simulink model "ThreeDOF_Rocket_Simulator_v2"  (R2023b)
settings: Solver=VariableStepAuto  StartTime=0.0  StopTime=100  RelTol=1e-3
libraries: shared3dof x1, simulink x1
settings Model: PacingRate=0.500000  Creator=giuse  LastModifiedBy=giuse
settings OptimizationCC: ReuseModelBlockBuffer=off
settings DebuggingCC: UnconnectedInputMsg=warning  UnconnectedOutputMsg=warning  UnconnectedLineMsg=warning
settings ModelReferenceCC: EnableRefExpFcnMdlSchedulingChecks=on
settings RTWCC: DLArmComputeVersion=19.05

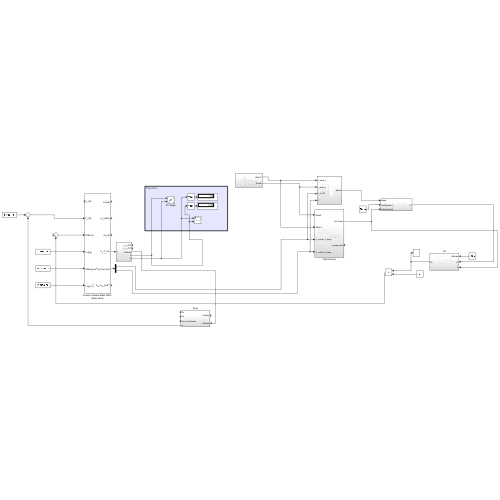
[thumbnail: Simulink's stored preview of the top-level diagram]
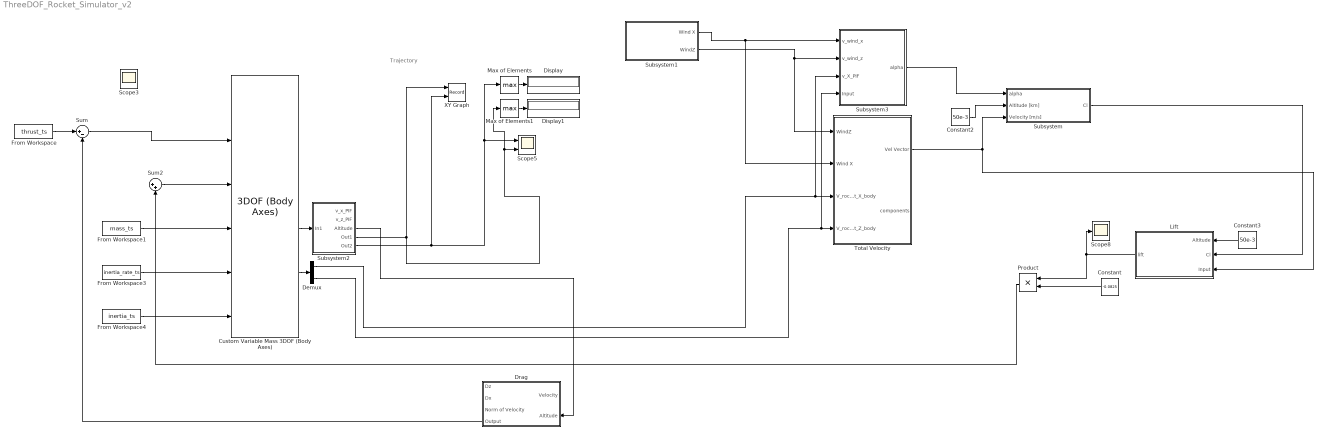
== system ThreeDOF_Rocket_Simulator_v2 ==
  note: Trajectory
  Constant : Constant  Value=-0.0825  VectorParams1D=off
  Constant2 : Constant  Value=50e-3
  Constant3 : Constant  Value=50e-3
  Custom Variable Mass 3DOF (Body Axes) : shared3dof/3DOF (Body Axes)  units=Metric (MKS)  mtype=Custom Variable  v_ini=0  theta_ini=pi  alpha_ini=pi/2  pos_ini=[0 0]  q_ini=0  mass=1.0  mass_e=0.5  mass_f=3.0  Iyy=1.0  Iyy_e=0.5  Iyy_f=3.0  g_in=Internal  g=9.81  vre_flag=off  abi_flag=off  aMode=0  vel_statename=''  theta_statename=''  pos_statename=''  q_statename=''  mass_statename=''
  Demux : Demux  Outputs=2
  Display : Display
  Display1 : Display
  Drag : Subsystem
  From Workspace : FromWorkspace  VariableName=thrust_ts
  From Workspace1 : FromWorkspace  VariableName=mass_ts
  From Workspace3 : FromWorkspace  VariableName=inertia_rate_ts
  From Workspace4 : FromWorkspace  VariableName=inertia_ts
  Lift : Subsystem
  Max of Elements : MinMax  Function=max
  Max of Elements1 : MinMax  Function=max
  Product : Product
  Scope5 : Scope  NumInputPorts=2
  Scope8 : Scope
  Subsystem : Subsystem
  Subsystem1 : Subsystem
  Subsystem2 : Subsystem
  Subsystem3 : Subsystem
  Sum : Sum  Inputs=|+-
  Sum2 : Sum  Inputs=|++
  Total Velocity : Subsystem
  XY Graph : Record  FileSettingsInternal="{\"entries\":[{\"content\":{\"excelSettings\":{\"content\":{},\"type\":\"Streamout.ExcelSettings\"}},\"type\":\"Streamout.FileSettingStorage\",\"uuid\":\"\"}],\"packageUris\":[\"http:\\/\\/schema.mathworks.com\\/mf0\\/streamout_blocks\\/R2020a\"],\"version\":\"1.0\"}"  Layout=[1 1]  SignalsInternal="{\"entries\":[{\"content\":{\"signals\":[{\"content\":{\"blockPath\":[],\"dimensions\":[1],\"domain\":\"\",\"lineColor\":\"#ff6929\",\"plots\":[1],\"port\":1,\"sid\":[\"\"],\"signalID\":744,\"signalName\":\"Subsystem2:4\"},\"type\":\"RecordBlkView.Signal\",\"uuid\":\"\"},{\"content\":{\"blockPath\":[],\"dimensions\":[1],\"domain\":\"\",\"lineColor\":\"#b746ff\",\"plots\":[1],\"port\":2,\"sid\":[\"\"],\"signalID\":748,\"signalName\":\"Subsystem2:5\"},\"type\":\"RecordBlkView.Signal\",\"uuid\":\"\"}]},\"type\":\"RecordBlkView.InputSignals\",\"uuid\":\"\"}],\"packageUris\":[\"http:\\/\\/schema.mathworks.com\\/mf0\\/streamout_blocks\\/R2020a\"],\"version\":\"1.0\"}"  VisualizationBindings="{\"xyplotplugin\":{\"info\":[{\"series\":[{\"bindingParametersList\":[{\"parameter\":\"X-Axis\",\"signalID\":748,\"signalName\":\"Subsystem2:5\"},{\"parameter\":\"Y-Axis\",\"signalID\":744,\"signalName\":\"Subsystem2:4\"}],\"seriesID\":7790}],\"subplotID\":1}]}}"  CompatibilityTag=XY
  Scope3 : Scope
  wires:
  From Workspace1/1 -> Custom Variable Mass 3DOF (Body Axes)/4
  From Workspace3/1 -> Custom Variable Mass 3DOF (Body Axes)/5
  From Workspace4/1 -> Custom Variable Mass 3DOF (Body Axes)/6
  From Workspace/1 -> Sum/1
  Sum/1 -> Custom Variable Mass 3DOF (Body Axes)/2
  Subsystem1/1(Wind X) -> Total Velocity/2(Wind X), Subsystem3/1(v_wind_x)
  Subsystem1/2(WindZ) -> Total Velocity/1(WindZ), Subsystem3/2(v_wind_z)
  Constant/1 -> Product/2
  Sum2/1 -> Custom Variable Mass 3DOF (Body Axes)/3
  Subsystem/1(Cl) -> Lift/2(Cl)
  Custom Variable Mass 3DOF (Body Axes)/4 -> Subsystem2/1(In1)
  Custom Variable Mass 3DOF (Body Axes)/5 -> Demux/1
  Total Velocity/1(Vel Vector) -> Lift/3(Input), Subsystem/3(Velocity [m/s])
  Demux/1 -> Total Velocity/3(V_rocket_X_body), Subsystem3/3(v_X_PIF)
  Demux/2 -> Total Velocity/4(V_rocket_Z_body), Subsystem3/4(Input)
  Subsystem2/4(Out1) -> Max of Elements1/1, Scope5/2, XY Graph/1
  Subsystem2/5(Out2) -> Max of Elements/1, Scope5/1, XY Graph/2
  Lift/1(lift) -> Product/1, Scope8/1
  Product/1 -> Sum2/2
  Constant2/1 -> Subsystem/2(Altitude [km])
  Constant3/1 -> Lift/1(Altitude)
  Subsystem2/3(Altitude) -> Drag/2(Altitude)
  Max of Elements/1 -> Display/1
  Max of Elements1/1 -> Display1/1
  Subsystem3/1(alpha) -> Subsystem/1(alpha)
  Drag/4(Output) -> Sum/2

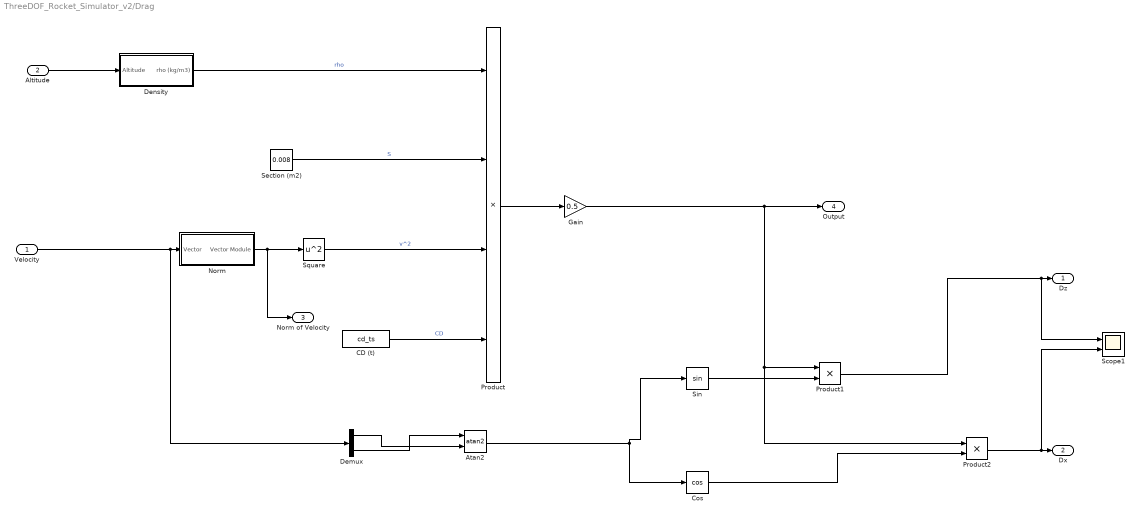
== system ThreeDOF_Rocket_Simulator_v2/Drag ==
  Velocity : Inport
  Altitude : Inport  Port=2
  Atan2 : Trigonometry  Operator=atan2
  CD (t) : FromWorkspace  VariableName=cd_ts
  Cos : Trigonometry  Operator=cos
  Demux : Demux  Outputs=2
  Density : Subsystem
  Gain : Gain  Gain=0.5
  Norm : Subsystem
  Product : Product  Inputs=4
  Product1 : Product
  Product2 : Product
  Scope1 : Scope  NumInputPorts=2
  Section (m2) : Constant  Value=0.008
  Sin : Trigonometry
  Square : Math  Operator=square
  Dz : Outport
  Dx : Outport  Port=2
  Norm of Velocity : Outport  Port=3
  Output : Outport  Port=4
  wires:
  Velocity/1 -> Demux/1, Norm/1(Vector)
  Altitude/1 -> Density/1(Altitude)
  Norm/1(Vector Module) -> Norm of Velocity/1, Square/1
  Density/1(rho (kg/m3)) -> Product/1  "rho"
  Section (m2)/1 -> Product/2  "S"
  Square/1 -> Product/3  "v^2"
  Product/1 -> Gain/1
  CD (t)/1 -> Product/4  "CD"
  Sin/1 -> Product1/2
  Gain/1 -> Output/1, Product2/1, Product1/1
  Cos/1 -> Product2/2
  Product2/1 -> Scope1/2, Dx/1
  Product1/1 -> Scope1/1, Dz/1
  Atan2/1 -> Sin/1, Cos/1
  Demux/2 -> Atan2/1
  Demux/1 -> Atan2/2

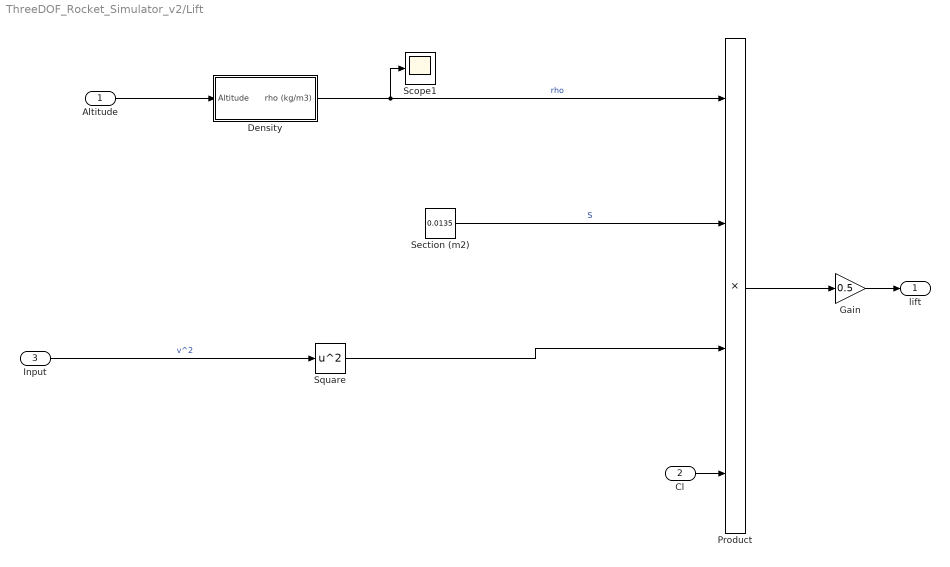
== system ThreeDOF_Rocket_Simulator_v2/Lift ==
  Altitude : Inport
  Cl : Inport  Port=2
  Input : Inport  Port=3
  Density : Subsystem
  Gain : Gain  Gain=0.5
  Product : Product  Inputs=4
  Scope1 : Scope
  Section (m2) : Constant  Value=0.0135
  Square : Math  Operator=square
  lift : Outport
  wires:
  Altitude/1 -> Density/1(Altitude)
  Density/1(rho (kg/m3)) -> Scope1/1, Product/1  "rho"
  Section (m2)/1 -> Product/2  "S"
  Product/1 -> Gain/1
  Cl/1 -> Product/4
  Input/1 -> Square/1  "v^2"
  Square/1 -> Product/3
  Gain/1 -> lift/1

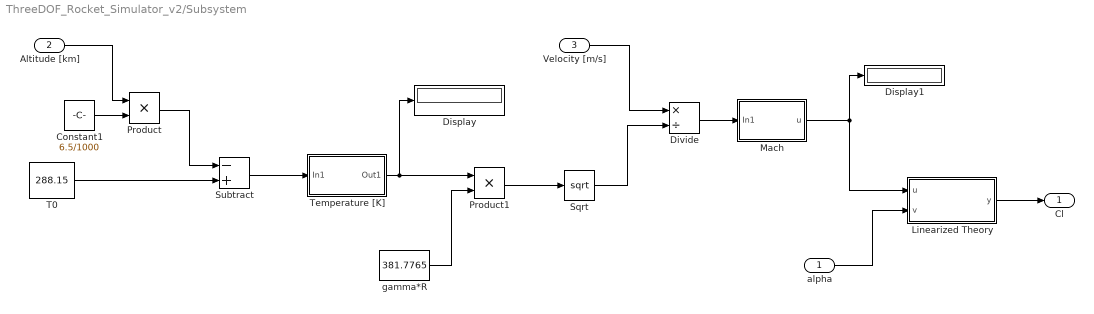
== system ThreeDOF_Rocket_Simulator_v2/Subsystem ==
  alpha : Inport
  Altitude [km] : Inport  Port=2
  Velocity [m/s] : Inport  Port=3
  Constant1 : Constant  Value=6.5/1000
  Display : Display
  Display1 : Display
  Divide : Product  Inputs=*/
  Linearized Theory : MATLAB Function  TreatAsAtomicUnit=on
  Mach : Subsystem
  Product : Product
  Product1 : Product
  Sqrt : Sqrt
  Subtract : Sum  Inputs=-+
  T0 : Constant  Value=288.15
  Temperature [K] : Subsystem
  gamma*R : Constant  Value=381.7765
  Cl : Outport
  wires:
  Constant1/1 -> Product/2
  Temperature [K]/1(Out1) -> Display/1, Product1/1
  T0/1 -> Subtract/2
  Subtract/1 -> Temperature [K]/1(In1)
  Mach/1(u) -> Display1/1, Linearized Theory/1(u)
  Divide/1 -> Mach/1(In1)
  Sqrt/1 -> Divide/2
  Product/1 -> Subtract/1
  gamma*R/1 -> Product1/2
  Velocity [m/s]/1 -> Divide/1
  Product1/1 -> Sqrt/1
  alpha/1 -> Linearized Theory/2(v)
  Linearized Theory/1(y) -> Cl/1
  Altitude [km]/1 -> Product/1

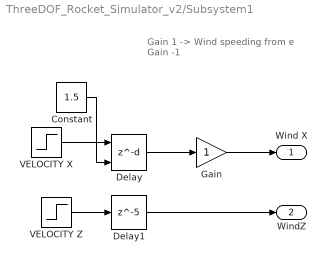
== system ThreeDOF_Rocket_Simulator_v2/Subsystem1 ==
  note: Gain 1 -> Wind speeding from e
      | Gain -1
  Constant : Constant  Value=1.5
  Delay : Delay  DelayLengthSource=Input port  DelayLength=1  DelayLengthUpperLimit=5  SampleTime=1
      settings: InputPortMap=u0,p1
  Delay1 : Delay  DelayLength=5  SampleTime=1
  Gain : Gain
  VELOCITY X : Step  Time=0.001  After=4  SampleTime=0
  VELOCITY Z : Step  Time=0  After=0  SampleTime=0
  Wind X : Outport
  WindZ : Outport  Port=2
  wires:
  Delay1/1 -> WindZ/1
  VELOCITY Z/1 -> Delay1/1
  Delay/1 -> Gain/1
  VELOCITY X/1 -> Delay/1
  Gain/1 -> Wind X/1
  Constant/1 -> Delay/2

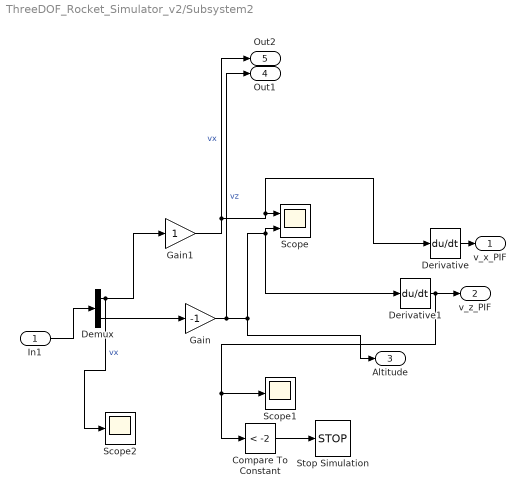
== system ThreeDOF_Rocket_Simulator_v2/Subsystem2 ==
  In1 : Inport
  Compare To Constant : simulink/Logic and Bit Operations/Compare To Constant  relop=<  const=-2  OutDataTypeStr=boolean
  Demux : Demux  Outputs=2
  Derivative : Derivative
  Derivative1 : Derivative
  Gain : Gain  Gain=-1
  Gain1 : Gain
  Scope : Scope  NumInputPorts=2
  Scope1 : Scope
  Scope2 : Scope
  Stop Simulation : Stop
  v_x_PIF : Outport
  v_z_PIF : Outport  Port=2
  Altitude : Outport  Port=3
  Out1 : Outport  Port=4
  Out2 : Outport  Port=5
  wires:
  Demux/2 -> Gain/1
  Gain/1 -> Out1/1, Altitude/1, Derivative1/1, Scope/2  "vz"
  In1/1 -> Demux/1
  Demux/1 -> Scope2/1, Gain1/1  "vx"
  Gain1/1 -> Out2/1, Derivative/1, Scope/1  "vx"
  Derivative1/1 -> Compare To Constant/1, Scope1/1, v_z_PIF/1
  Compare To Constant/1 -> Stop Simulation/1
  Derivative/1 -> v_x_PIF/1

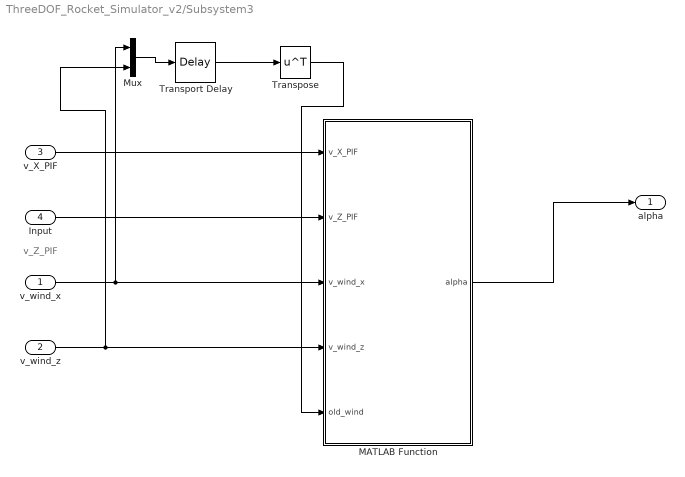
== system ThreeDOF_Rocket_Simulator_v2/Subsystem3 ==
  note: v_Z_PIF
  v_wind_x : Inport
  v_wind_z : Inport  Port=2
  v_X_PIF : Inport  Port=3
  Input : Inport  Port=4
  MATLAB Function : MATLAB Function  TreatAsAtomicUnit=on
  Mux : Mux  Inputs=2
  Transport Delay : TransportDelay  DelayTime=0.005
  Transpose : Math  Operator=transpose
  alpha : Outport
  wires:
  v_wind_x/1 -> MATLAB Function/3(v_wind_x), Mux/1
  MATLAB Function/1(alpha) -> alpha/1
  Transpose/1 -> MATLAB Function/5(old_wind)
  Mux/1 -> Transport Delay/1
  Transport Delay/1 -> Transpose/1
  Input/1 -> MATLAB Function/2(v_Z_PIF)
  v_wind_z/1 -> MATLAB Function/4(v_wind_z), Mux/2
  v_X_PIF/1 -> MATLAB Function/1(v_X_PIF)

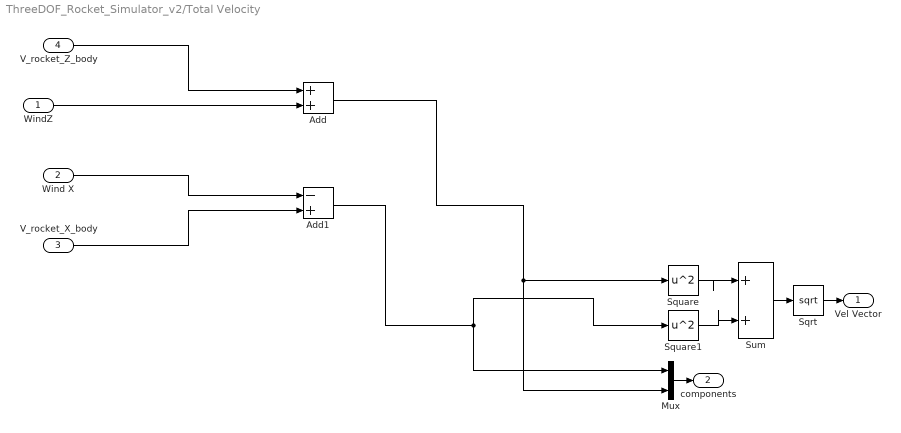
== system ThreeDOF_Rocket_Simulator_v2/Total Velocity ==
  WindZ : Inport
  Wind X : Inport  Port=2
  V_rocket_X_body : Inport  Port=3
  V_rocket_Z_body : Inport  Port=4
  Add : Sum
  Add1 : Sum  Inputs=-+
  Mux : Mux  Inputs=2
  Sqrt : Sqrt
  Square : Math  Operator=square
  Square1 : Math  Operator=square
  Sum : Sum  Inputs=|++|
  Vel Vector : Outport
  components : Outport  Port=2
  wires:
  Wind X/1 -> Add1/1
  Add1/1 -> Square1/1, Mux/1
  Add/1 -> Square/1, Mux/2
  WindZ/1 -> Add/2
  V_rocket_Z_body/1 -> Add/1
  V_rocket_X_body/1 -> Add1/2
  Square/1 -> Sum/1
  Square1/1 -> Sum/2
  Sum/1 -> Sqrt/1
  Sqrt/1 -> Vel Vector/1
  Mux/1 -> components/1

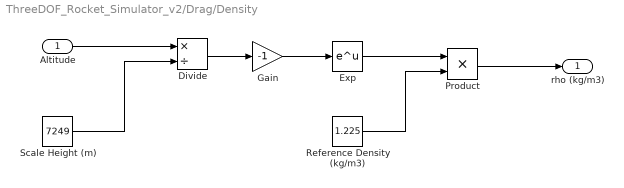
== system ThreeDOF_Rocket_Simulator_v2/Drag/Density ==
  Altitude : Inport
  Divide : Product  Inputs=*/
  Exp : Math
  Gain : Gain  Gain=-1
  Product : Product
  Reference Density (kg/m3) : Constant  Value=1.225
  Scale Height (m) : Constant  Value=7249
  rho (kg/m3) : Outport
  wires:
  Altitude/1 -> Divide/1
  Scale Height (m)/1 -> Divide/2
  Divide/1 -> Gain/1
  Gain/1 -> Exp/1
  Exp/1 -> Product/1
  Reference Density (kg/m3)/1 -> Product/2
  Product/1 -> rho (kg/m3)/1

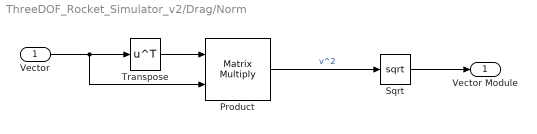
== system ThreeDOF_Rocket_Simulator_v2/Drag/Norm ==
  Vector : Inport
  Product : Product  Multiplication=Matrix(*)
  Sqrt : Sqrt
  Transpose : Math  Operator=transpose
  Vector Module : Outport
  wires:
  Vector/1 -> Product/2, Transpose/1
  Product/1 -> Sqrt/1  "v^2"
  Sqrt/1 -> Vector Module/1
  Transpose/1 -> Product/1

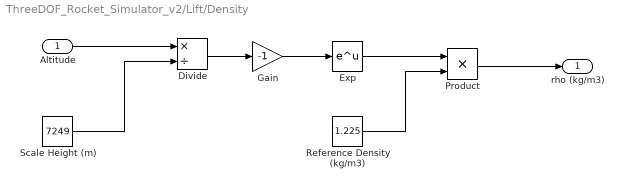
== system ThreeDOF_Rocket_Simulator_v2/Lift/Density ==
  Altitude : Inport
  Divide : Product  Inputs=*/
  Exp : Math
  Gain : Gain  Gain=-1
  Product : Product
  Reference Density (kg/m3) : Constant  Value=1.225
  Scale Height (m) : Constant  Value=7249
  rho (kg/m3) : Outport
  wires:
  Altitude/1 -> Divide/1
  Scale Height (m)/1 -> Divide/2
  Divide/1 -> Gain/1
  Gain/1 -> Exp/1
  Exp/1 -> Product/1
  Reference Density (kg/m3)/1 -> Product/2
  Product/1 -> rho (kg/m3)/1

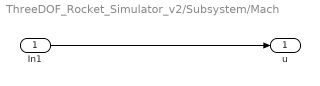
== system ThreeDOF_Rocket_Simulator_v2/Subsystem/Mach ==
  In1 : Inport
  u : Outport
  wires:
  In1/1 -> u/1

== system ThreeDOF_Rocket_Simulator_v2/Subsystem/Temperature [K] ==
  In1 : Inport
  Out1 : Outport
  wires:
  In1/1 -> Out1/1

== matlab function ThreeDOF_Rocket_Simulator_v2/Subsystem3/MATLAB Function ==
  data: v_X_PIF input; alpha output; v_Z_PIF input; v_wind_x input; v_wind_z input; old_wind input
function alpha  = fcn(v_X_PIF,v_Z_PIF,v_wind_x,v_wind_z,old_wind)

%Calculation of the angle of attack
% having the information about velocity in PIF we need to evaluate whether
% the rocket is flying parallel or not to the stream of the wind. In fact
% if not it will start correcting the angle of attack, in the other case
% the angle the attack will be set to zero
V_PIF = [v_X_PIF,v_Z_PIF];
V_WIND = [v_wind_x,v_wind_z];
old_wind;
norm(old_wind,2);
norm(V_WIND,2);
if norm(old_wind,2)-norm(V_WIND,2) ~= 0
%calculation of the angle between velocity of the rocket in PIF MENUS wind and versor k
%if this angle is near to zero
disp("here debug")
  alpha = 1.75*pi/180  %value that we need to feed into cl subsystem
else 
    alpha = 0
end

disp("-------------")

== matlab function ThreeDOF_Rocket_Simulator_v2/Subsystem/Linearized Theory ==
  data: u input; y output; v input
function y = fcn(u,v)
% First method, linearized theory for a thin plate
% if u<1
%     y = ((2*pi*(v*2*pi)/360)./(sqrt(1-u.^2)))*(13500/(2*pi*(52)^2).*2)
%     y= 1.648
% else
%     y= 4*(4*(v*pi/180))./(sqrt(u.^2-1)+2*(v*pi/180))
% 
% end


if v==0
    y =0
else 
    y=0.435
end
